simulink model "L0304"  (Simulink 10.2)
settings: Solver=ode45  StartTime=0.0  StopTime=20  MaxStep=0.01  RelTol=1e-3
libraries: simulink x4
settings Model: Creator=Ranci  LastModifiedBy=Ranci
settings DataIOCC: SaveFormat=Dataset  SignalLoggingSaveFormat=Dataset  ReturnWorkspaceOutputs=on
settings OptimizationCC: LifeSpan=auto
settings DebuggingCC: UnderspecifiedInitializationDetection=Simplified  MergeDetectMultiDrivingBlocksExec=error  FcnCallInpInsideContextMsg=error  SFUnexpectedBacktrackingDiag=error  SFNoUnconditionalDefaultTransitionDiag=error  SFExecutionAtInitializationDiag=warning  ArithmeticOperatorsInVariantConditions=error
settings HardwareCC: ProdBitPerPointer=64  ProdBitPerSizeT=64  ProdBitPerPtrDiffT=64  ProdLargestAtomicFloat=Float  ProdIntDivRoundTo=Zero  ProdEndianess=LittleEndian  ProdWordSize=64  ProdHWDeviceType=Intel->x86-64 (Windows64)
settings ModelReferenceCC: PropagateSignalLabelsOutOfModel=on
settings SFSimCC: SimUseLocalCustomCode=on  CustomCodeUndefinedFunction=FilterOut
settings RTWCC: RTWUseLocalCustomCode=on
settings CodeAppCC: StateflowObjectComments=off
settings GRTTargetCC: TargetLangStandard=C99 (ISO)  CombineOutputUpdateFcns=on  GRTInterface=off
settings ConfigComp: CovMetricSettings=dwe  CovSaveCumulativeToWorkspaceVar=off  CovSaveSingleToWorkspaceVar=off  CovExternalEMLEnable=on

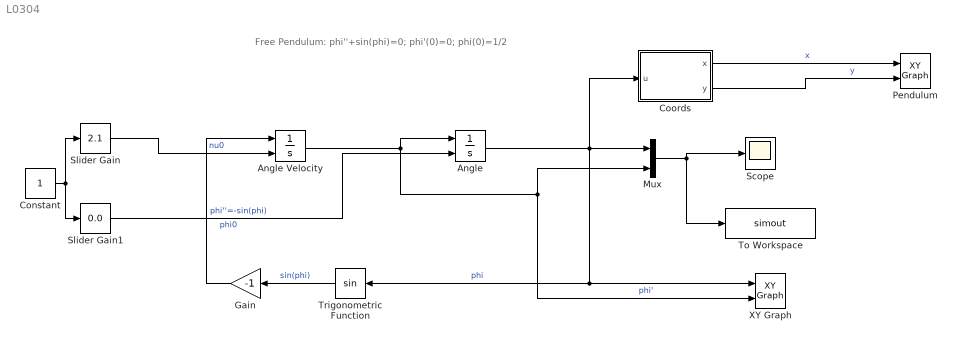
== system L0304 ==
  note: Free Pendulum: phi''+sin(phi)=0; phi'(0)=0; phi(0)=1/2
  Angle : Integrator  InitialConditionSource=external  InitialCondition=1/2
  Angle Velocity : Integrator  InitialConditionSource=external
  Constant : Constant
  Coords : MATLAB Function  TreatAsAtomicUnit=on
  Gain : Gain  Gain=-1
  Mux : Mux  Inputs=2
  Pendulum : simulink/Sinks/XY Graph  xmin=-1  xmax=1  ymin=-1  ymax=1  st=-1
  Scope : Scope
  Slider Gain : simulink/Math Operations/Slider Gain  gain=2.1  low=0  high=3
  Slider Gain1 : simulink/Math Operations/Slider Gain  gain=0.0  low=0  high=6
  To Workspace : ToWorkspace  VariableName=simout  SaveFormat=Structure With Time  SampleTime=-1
  Trigonometric Function : Trigonometry
  XY Graph : simulink/Sinks/XY Graph  xmin=-6  xmax=6  ymin=-6  ymax=6  st=-1
  wires:
  Gain/1 -> Angle Velocity/1  "phi''=-sin(phi)"
  Angle Velocity/1 -> Angle/1, XY Graph/2, Mux/2  "phi'"
  Trigonometric Function/1 -> Gain/1  "sin(phi)"
  Angle/1 -> Coords/1(u), Mux/1, Trigonometric Function/1, XY Graph/1  "phi"
  Mux/1 -> Scope/1, To Workspace/1
  Slider Gain/1 -> Angle Velocity/2  "nu0"
  Slider Gain1/1 -> Angle/2  "phi0"
  Coords/1(x) -> Pendulum/1  "x"
  Coords/2(y) -> Pendulum/2  "y"
  Constant/1 -> Slider Gain/1, Slider Gain1/1

== matlab function Coords ==
  data: x output double; u input double; y output double
function [x,y] = fcn(u)
L = 1;       % длина нити
x = L * sin(u);
y = -L * cos(u);
